simulink library "xrbsMath_r3"  (Simulink 5.0)
undefined symbols (not defined in the file or in its folder): num_width
libraries: xbsIndex_r3 x775, xrbsMath_r3 x16
(part 5 of 8)

== system xrbsMath_r3/CORDIC LOG/CORDIC Fine Angle PE/CORDIC PE4 ==
  note: X = x + y if y < 0, otherwise
      |    = x - y
      | Y = y + x if y < 0, otherwise
      |    = y - x
      | Z = z - atanh(1/2^i) if y < 0, otherwise
      |    = z + atanh(1/2^i)
  x : Inport
  y : Inport  Port=2
  z : Inport  Port=3
  AddSub : xbsIndex_r3/AddSub  mode=Addition or Subtraction  precision=User Defined  arith_type="Signed  (2's comp)"  n_bits=pe_nbits  bin_pt=pe_binpt  quantization=Truncate  overflow=Wrap  latency=pipeline  explicit_period=off  period=1  en=off  dbl_ovrd=off  use_core=on  pipeline=off  use_rpm=off  gen_core=on
      settings: xl_area=[7 14 0 14 0 0 0]
  AddSub1 : xbsIndex_r3/AddSub  mode=Addition or Subtraction  precision=User Defined  arith_type="Signed  (2's comp)"  n_bits=pe_nbits  bin_pt=pe_binpt  quantization=Truncate  overflow=Wrap  latency=pipeline  explicit_period=off  period=1  en=off  dbl_ovrd=off  use_core=on  pipeline=off  use_rpm=off  gen_core=on
      settings: xl_area=[7 14 0 14 0 0 0]
  AddSub2 : xbsIndex_r3/AddSub  mode=Addition or Subtraction  precision=User Defined  arith_type="Signed  (2's comp)"  n_bits=pe_nbits  bin_pt=pe_binpt  quantization=Truncate  overflow=Wrap  latency=pipeline  explicit_period=off  period=1  en=off  dbl_ovrd=off  use_core=on  pipeline=off  use_rpm=off  gen_core=on
      settings: xl_area=[0, 0, 0, 0, 0, 0, 0]
  Constant : xbsIndex_r3/Constant  const=atanh(1/2^ii)  arith_type="Signed  (2's comp)"  n_bits=pe_nbits  bin_pt=pe_binpt  explicit_period=off  period=1  dbl_ovrd=off
  Inverter : xbsIndex_r3/Inverter  latency=0  explicit_period=off  period=1  en=off  dbl_ovrd=off
      settings: xl_area=[1 0 0 1 0 0 0]
  Shift : xbsIndex_r3/Shift  shift_dir=Right  shift_bits=ii  precision=User Defined  arith_type="Signed  (2's comp)"  n_bits=pe_nbits  bin_pt=pe_binpt  quantization=Truncate  overflow=Wrap  latency=0  explicit_period=off  period=1  en=off  dbl_ovrd=off
      settings: xl_area=[0 0 0 0 0 0 0]
  Shift1 : xbsIndex_r3/Shift  shift_dir=Right  shift_bits=ii  precision=User Defined  arith_type="Signed  (2's comp)"  n_bits=pe_nbits  bin_pt=pe_binpt  quantization=Truncate  overflow=Wrap  latency=0  explicit_period=off  period=1  en=off  dbl_ovrd=off
      settings: xl_area=[0 0 0 0 0 0 0]
  Slice : xbsIndex_r3/Slice  mode=Upper Bit Location + Width  nbits=1  bit1=0  base1=MSB of Input  bit0=0  base0=LSB of Input  boolean_output=on  explicit_period=off  period=1  dbl_ovrd=off
  X : Outport
  Y : Outport  Port=2
  Z : Outport  Port=3
  wires:
  Constant/1 -> AddSub2/2
  AddSub2/1 -> Z/1
  z/1 -> AddSub2/1
  Slice/1 -> AddSub2/3, Inverter/1
  Shift1/1 -> AddSub/2
  Shift/1 -> AddSub1/2
  AddSub1/1 -> Y/1
  AddSub/1 -> X/1
  y/1 -> Slice/1, Shift1/1, AddSub1/1
  x/1 -> Shift/1, AddSub/1
  Inverter/1 -> AddSub/3, AddSub1/3

== system xrbsMath_r3/CORDIC LOG/CORDIC Fine Angle PE/CORDIC PE5 ==
  note: X = x + y if y < 0, otherwise
      |    = x - y
      | Y = y + x if y < 0, otherwise
      |    = y - x
      | Z = z - atanh(1/2^i) if y < 0, otherwise
      |    = z + atanh(1/2^i)
  x : Inport
  y : Inport  Port=2
  z : Inport  Port=3
  AddSub : xbsIndex_r3/AddSub  mode=Addition or Subtraction  precision=User Defined  arith_type="Signed  (2's comp)"  n_bits=pe_nbits  bin_pt=pe_binpt  quantization=Truncate  overflow=Wrap  latency=pipeline  explicit_period=off  period=1  en=off  dbl_ovrd=off  use_core=on  pipeline=off  use_rpm=off  gen_core=on
      settings: xl_area=[7 14 0 14 0 0 0]
  AddSub1 : xbsIndex_r3/AddSub  mode=Addition or Subtraction  precision=User Defined  arith_type="Signed  (2's comp)"  n_bits=pe_nbits  bin_pt=pe_binpt  quantization=Truncate  overflow=Wrap  latency=pipeline  explicit_period=off  period=1  en=off  dbl_ovrd=off  use_core=on  pipeline=off  use_rpm=off  gen_core=on
      settings: xl_area=[7 14 0 14 0 0 0]
  AddSub2 : xbsIndex_r3/AddSub  mode=Addition or Subtraction  precision=User Defined  arith_type="Signed  (2's comp)"  n_bits=pe_nbits  bin_pt=pe_binpt  quantization=Truncate  overflow=Wrap  latency=pipeline  explicit_period=off  period=1  en=off  dbl_ovrd=off  use_core=on  pipeline=off  use_rpm=off  gen_core=on
      settings: xl_area=[0, 0, 0, 0, 0, 0, 0]
  Constant : xbsIndex_r3/Constant  const=atanh(1/2^ii)  arith_type="Signed  (2's comp)"  n_bits=pe_nbits  bin_pt=pe_binpt  explicit_period=off  period=1  dbl_ovrd=off
  Inverter : xbsIndex_r3/Inverter  latency=0  explicit_period=off  period=1  en=off  dbl_ovrd=off
      settings: xl_area=[1 0 0 1 0 0 0]
  Shift : xbsIndex_r3/Shift  shift_dir=Right  shift_bits=ii  precision=User Defined  arith_type="Signed  (2's comp)"  n_bits=pe_nbits  bin_pt=pe_binpt  quantization=Truncate  overflow=Wrap  latency=0  explicit_period=off  period=1  en=off  dbl_ovrd=off
      settings: xl_area=[0 0 0 0 0 0 0]
  Shift1 : xbsIndex_r3/Shift  shift_dir=Right  shift_bits=ii  precision=User Defined  arith_type="Signed  (2's comp)"  n_bits=pe_nbits  bin_pt=pe_binpt  quantization=Truncate  overflow=Wrap  latency=0  explicit_period=off  period=1  en=off  dbl_ovrd=off
      settings: xl_area=[0 0 0 0 0 0 0]
  Slice : xbsIndex_r3/Slice  mode=Upper Bit Location + Width  nbits=1  bit1=0  base1=MSB of Input  bit0=0  base0=LSB of Input  boolean_output=on  explicit_period=off  period=1  dbl_ovrd=off
  X : Outport
  Y : Outport  Port=2
  Z : Outport  Port=3
  wires:
  Constant/1 -> AddSub2/2
  AddSub2/1 -> Z/1
  z/1 -> AddSub2/1
  Slice/1 -> AddSub2/3, Inverter/1
  Shift1/1 -> AddSub/2
  Shift/1 -> AddSub1/2
  AddSub1/1 -> Y/1
  AddSub/1 -> X/1
  y/1 -> Slice/1, Shift1/1, AddSub1/1
  x/1 -> Shift/1, AddSub/1
  Inverter/1 -> AddSub/3, AddSub1/3

== system xrbsMath_r3/CORDIC LOG/CORDIC Fine Angle PE/CORDIC PE6 ==
  note: X = x + y if y < 0, otherwise
      |    = x - y
      | Y = y + x if y < 0, otherwise
      |    = y - x
      | Z = z - atanh(1/2^i) if y < 0, otherwise
      |    = z + atanh(1/2^i)
  x : Inport
  y : Inport  Port=2
  z : Inport  Port=3
  AddSub : xbsIndex_r3/AddSub  mode=Addition or Subtraction  precision=User Defined  arith_type="Signed  (2's comp)"  n_bits=pe_nbits  bin_pt=pe_binpt  quantization=Truncate  overflow=Wrap  latency=pipeline  explicit_period=off  period=1  en=off  dbl_ovrd=off  use_core=on  pipeline=off  use_rpm=off  gen_core=on
      settings: xl_area=[7 14 0 14 0 0 0]
  AddSub1 : xbsIndex_r3/AddSub  mode=Addition or Subtraction  precision=User Defined  arith_type="Signed  (2's comp)"  n_bits=pe_nbits  bin_pt=pe_binpt  quantization=Truncate  overflow=Wrap  latency=pipeline  explicit_period=off  period=1  en=off  dbl_ovrd=off  use_core=on  pipeline=off  use_rpm=off  gen_core=on
      settings: xl_area=[7 14 0 14 0 0 0]
  AddSub2 : xbsIndex_r3/AddSub  mode=Addition or Subtraction  precision=User Defined  arith_type="Signed  (2's comp)"  n_bits=pe_nbits  bin_pt=pe_binpt  quantization=Truncate  overflow=Wrap  latency=pipeline  explicit_period=off  period=1  en=off  dbl_ovrd=off  use_core=on  pipeline=off  use_rpm=off  gen_core=on
      settings: xl_area=[0, 0, 0, 0, 0, 0, 0]
  Constant : xbsIndex_r3/Constant  const=atanh(1/2^ii)  arith_type="Signed  (2's comp)"  n_bits=pe_nbits  bin_pt=pe_binpt  explicit_period=off  period=1  dbl_ovrd=off
  Inverter : xbsIndex_r3/Inverter  latency=0  explicit_period=off  period=1  en=off  dbl_ovrd=off
      settings: xl_area=[1 0 0 1 0 0 0]
  Shift : xbsIndex_r3/Shift  shift_dir=Right  shift_bits=ii  precision=User Defined  arith_type="Signed  (2's comp)"  n_bits=pe_nbits  bin_pt=pe_binpt  quantization=Truncate  overflow=Wrap  latency=0  explicit_period=off  period=1  en=off  dbl_ovrd=off
      settings: xl_area=[0 0 0 0 0 0 0]
  Shift1 : xbsIndex_r3/Shift  shift_dir=Right  shift_bits=ii  precision=User Defined  arith_type="Signed  (2's comp)"  n_bits=pe_nbits  bin_pt=pe_binpt  quantization=Truncate  overflow=Wrap  latency=0  explicit_period=off  period=1  en=off  dbl_ovrd=off
      settings: xl_area=[0 0 0 0 0 0 0]
  Slice : xbsIndex_r3/Slice  mode=Upper Bit Location + Width  nbits=1  bit1=0  base1=MSB of Input  bit0=0  base0=LSB of Input  boolean_output=on  explicit_period=off  period=1  dbl_ovrd=off
  X : Outport
  Y : Outport  Port=2
  Z : Outport  Port=3
  wires:
  Constant/1 -> AddSub2/2
  AddSub2/1 -> Z/1
  z/1 -> AddSub2/1
  Slice/1 -> AddSub2/3, Inverter/1
  Shift1/1 -> AddSub/2
  Shift/1 -> AddSub1/2
  AddSub1/1 -> Y/1
  AddSub/1 -> X/1
  y/1 -> Slice/1, Shift1/1, AddSub1/1
  x/1 -> Shift/1, AddSub/1
  Inverter/1 -> AddSub/3, AddSub1/3

== system xrbsMath_r3/CORDIC LOG/CORDIC Fine Angle PE/CORDIC PE7 ==
  note: X = x + y if y < 0, otherwise
      |    = x - y
      | Y = y + x if y < 0, otherwise
      |    = y - x
      | Z = z - atanh(1/2^i) if y < 0, otherwise
      |    = z + atanh(1/2^i)
  x : Inport
  y : Inport  Port=2
  z : Inport  Port=3
  AddSub : xbsIndex_r3/AddSub  mode=Addition or Subtraction  precision=User Defined  arith_type="Signed  (2's comp)"  n_bits=pe_nbits  bin_pt=pe_binpt  quantization=Truncate  overflow=Wrap  latency=pipeline  explicit_period=off  period=1  en=off  dbl_ovrd=off  use_core=on  pipeline=off  use_rpm=off  gen_core=on
      settings: xl_area=[7 14 0 14 0 0 0]
  AddSub1 : xbsIndex_r3/AddSub  mode=Addition or Subtraction  precision=User Defined  arith_type="Signed  (2's comp)"  n_bits=pe_nbits  bin_pt=pe_binpt  quantization=Truncate  overflow=Wrap  latency=pipeline  explicit_period=off  period=1  en=off  dbl_ovrd=off  use_core=on  pipeline=off  use_rpm=off  gen_core=on
      settings: xl_area=[7 14 0 14 0 0 0]
  AddSub2 : xbsIndex_r3/AddSub  mode=Addition or Subtraction  precision=User Defined  arith_type="Signed  (2's comp)"  n_bits=pe_nbits  bin_pt=pe_binpt  quantization=Truncate  overflow=Wrap  latency=pipeline  explicit_period=off  period=1  en=off  dbl_ovrd=off  use_core=on  pipeline=off  use_rpm=off  gen_core=on
      settings: xl_area=[0, 0, 0, 0, 0, 0, 0]
  Constant : xbsIndex_r3/Constant  const=atanh(1/2^ii)  arith_type="Signed  (2's comp)"  n_bits=pe_nbits  bin_pt=pe_binpt  explicit_period=off  period=1  dbl_ovrd=off
  Inverter : xbsIndex_r3/Inverter  latency=0  explicit_period=off  period=1  en=off  dbl_ovrd=off
      settings: xl_area=[1 0 0 1 0 0 0]
  Shift : xbsIndex_r3/Shift  shift_dir=Right  shift_bits=ii  precision=User Defined  arith_type="Signed  (2's comp)"  n_bits=pe_nbits  bin_pt=pe_binpt  quantization=Truncate  overflow=Wrap  latency=0  explicit_period=off  period=1  en=off  dbl_ovrd=off
      settings: xl_area=[0 0 0 0 0 0 0]
  Shift1 : xbsIndex_r3/Shift  shift_dir=Right  shift_bits=ii  precision=User Defined  arith_type="Signed  (2's comp)"  n_bits=pe_nbits  bin_pt=pe_binpt  quantization=Truncate  overflow=Wrap  latency=0  explicit_period=off  period=1  en=off  dbl_ovrd=off
      settings: xl_area=[0 0 0 0 0 0 0]
  Slice : xbsIndex_r3/Slice  mode=Upper Bit Location + Width  nbits=1  bit1=0  base1=MSB of Input  bit0=0  base0=LSB of Input  boolean_output=on  explicit_period=off  period=1  dbl_ovrd=off
  X : Outport
  Y : Outport  Port=2
  Z : Outport  Port=3
  wires:
  Constant/1 -> AddSub2/2
  AddSub2/1 -> Z/1
  z/1 -> AddSub2/1
  Slice/1 -> AddSub2/3, Inverter/1
  Shift1/1 -> AddSub/2
  Shift/1 -> AddSub1/2
  AddSub1/1 -> Y/1
  AddSub/1 -> X/1
  y/1 -> Slice/1, Shift1/1, AddSub1/1
  x/1 -> Shift/1, AddSub/1
  Inverter/1 -> AddSub/3, AddSub1/3

== system xrbsMath_r3/CORDIC LOG/CORDIC Fine Angle PE/CORDIC PE8 ==
  note: X = x + y if y < 0, otherwise
      |    = x - y
      | Y = y + x if y < 0, otherwise
      |    = y - x
      | Z = z - atanh(1/2^i) if y < 0, otherwise
      |    = z + atanh(1/2^i)
  x : Inport
  y : Inport  Port=2
  z : Inport  Port=3
  AddSub : xbsIndex_r3/AddSub  mode=Addition or Subtraction  precision=User Defined  arith_type="Signed  (2's comp)"  n_bits=pe_nbits  bin_pt=pe_binpt  quantization=Truncate  overflow=Wrap  latency=pipeline  explicit_period=off  period=1  en=off  dbl_ovrd=off  use_core=on  pipeline=off  use_rpm=off  gen_core=on
      settings: xl_area=[7 14 0 14 0 0 0]
  AddSub1 : xbsIndex_r3/AddSub  mode=Addition or Subtraction  precision=User Defined  arith_type="Signed  (2's comp)"  n_bits=pe_nbits  bin_pt=pe_binpt  quantization=Truncate  overflow=Wrap  latency=pipeline  explicit_period=off  period=1  en=off  dbl_ovrd=off  use_core=on  pipeline=off  use_rpm=off  gen_core=on
      settings: xl_area=[7 14 0 14 0 0 0]
  AddSub2 : xbsIndex_r3/AddSub  mode=Addition or Subtraction  precision=User Defined  arith_type="Signed  (2's comp)"  n_bits=pe_nbits  bin_pt=pe_binpt  quantization=Truncate  overflow=Wrap  latency=pipeline  explicit_period=off  period=1  en=off  dbl_ovrd=off  use_core=on  pipeline=off  use_rpm=off  gen_core=on
      settings: xl_area=[0, 0, 0, 0, 0, 0, 0]
  Constant : xbsIndex_r3/Constant  const=atanh(1/2^ii)  arith_type="Signed  (2's comp)"  n_bits=pe_nbits  bin_pt=pe_binpt  explicit_period=off  period=1  dbl_ovrd=off
  Inverter : xbsIndex_r3/Inverter  latency=0  explicit_period=off  period=1  en=off  dbl_ovrd=off
      settings: xl_area=[1 0 0 1 0 0 0]
  Shift : xbsIndex_r3/Shift  shift_dir=Right  shift_bits=ii  precision=User Defined  arith_type="Signed  (2's comp)"  n_bits=pe_nbits  bin_pt=pe_binpt  quantization=Truncate  overflow=Wrap  latency=0  explicit_period=off  period=1  en=off  dbl_ovrd=off
      settings: xl_area=[0 0 0 0 0 0 0]
  Shift1 : xbsIndex_r3/Shift  shift_dir=Right  shift_bits=ii  precision=User Defined  arith_type="Signed  (2's comp)"  n_bits=pe_nbits  bin_pt=pe_binpt  quantization=Truncate  overflow=Wrap  latency=0  explicit_period=off  period=1  en=off  dbl_ovrd=off
      settings: xl_area=[0 0 0 0 0 0 0]
  Slice : xbsIndex_r3/Slice  mode=Upper Bit Location + Width  nbits=1  bit1=0  base1=MSB of Input  bit0=0  base0=LSB of Input  boolean_output=on  explicit_period=off  period=1  dbl_ovrd=off
  X : Outport
  Y : Outport  Port=2
  Z : Outport  Port=3
  wires:
  Constant/1 -> AddSub2/2
  AddSub2/1 -> Z/1
  z/1 -> AddSub2/1
  Slice/1 -> AddSub2/3, Inverter/1
  Shift1/1 -> AddSub/2
  Shift/1 -> AddSub1/2
  AddSub1/1 -> Y/1
  AddSub/1 -> X/1
  y/1 -> Slice/1, Shift1/1, AddSub1/1
  x/1 -> Shift/1, AddSub/1
  Inverter/1 -> AddSub/3, AddSub1/3

== system xrbsMath_r3/CORDIC LOG/Quadrant Map/Co-ordinate Correction ==
  x : Inport
  Constant3 : xbsIndex_r3/Constant  const=0  arith_type=Unsigned  n_bits=1  bin_pt=0  explicit_period=off  period=1  dbl_ovrd=off
  Delay4 : xbsIndex_r3/Delay  latency=1  reg_retiming=off  explicit_period=off  period=1  en=off  accept_only_valid=off  init_zero=on  dbl_ovrd=off
      settings: xl_area=[6 12 0 0 0 0 0]
  Mux : xbsIndex_r3/Mux  inputs=2  precision=User Defined  arith_type="Signed  (2's comp)"  n_bits=pe_nbits  bin_pt=pe_binpt  quantization=Truncate  overflow=Wrap  latency=1  mux_type=off  explicit_period=off  period=1  en=off  dbl_ovrd=off  use_rpm=off  gen_core=on
      settings: xl_area=[6 12 0 12 0 0 0]
  Negate1 : xbsIndex_r3/Negate  precision=User Defined  arith_type="Signed  (2's comp)"  n_bits=pe_nbits  bin_pt=pe_binpt  quantization=Truncate  overflow=Wrap  latency=0  explicit_period=off  period=1  en=off  dbl_ovrd=off  use_core=on  use_rpm=off  gen_core=on
      settings: xl_area=[6 0 0 12 0 0 0]
  Reinterpret : xbsIndex_r3/Reinterpret  force_arith_type=off  arith_type="Signed  (2's comp)"  force_bin_pt=on  bin_pt=pe_nbits-1  force_valid=on
  Relational : xbsIndex_r3/Relational  mode=a=b  latency=1  explicit_period=off  period=1  en=off  dbl_ovrd=off
      settings: xl_area=[3 0 0 6 0 0 0]
  sgn(x) : xbsIndex_r3/Slice  mode=Upper Bit Location + Width  nbits=1  bit1=0  base1=MSB of Input  bit0=0  base0=LSB of Input  boolean_output=off  explicit_period=off  period=1  dbl_ovrd=off
  X : Outport
  sign_x : Outport  Port=2
  zero_detect : Outport  Port=3
  wires:
  Relational/1 -> zero_detect/1
  x/1 -> Delay4/1
  Constant3/1 -> Relational/2
  Reinterpret/1 -> X/1
  Mux/1 -> Reinterpret/1
  Negate1/1 -> Mux/3
  sgn(x)/1 -> sign_x/1, Mux/1
  Delay4/1 -> Relational/1, sgn(x)/1, Negate1/1, Mux/2

== system xrbsMath_r3/CORDIC LOG/Quadrant Map/Normalize X ==
  note: Normalizing X : The absolute value of X is shifted left till we have a 1
      | on the most significant bit and the number of shifts are recorded.
  abs : Inport
  cin : Inport  Port=2
  msb : Inport  Port=3
  Shift1 : Subsystem  mask(Normalize Shift Stage){num_bits=num_bits, bin_point=bin_point}
      mask prompts: num_bits "Number of Bits"; bin_point "Binary Point Position"
      mask init:
      | [bg,fg] = xlcmap('XBlock',0);
      | iPos = get_param(gcb,'Position');
      | iWidth=iPos(3)-iPos(1); iHeight=iPos(4)-iPos(2);
      | iCx=iWidth/2;
      | iCy=iHeight/2;
      | [logoX, logoY] = xlogo(iPos);
      mask Display:
      | patch([0 iWidth iWidth 0],[0 0 iHeight iHeight] , bg);
      | patch(logoX,logoY , fg);
      | port_label('input',1,'din');
      | port_label('input',2,'cin');
      | port_label('input',3,'msb');
      | port_label('output',1,'dout');
      | port_label('output',2,'sum');
      | port_label('output',3,'latch');
      | plot([0 0 iWidth iWidth 0], [0 iHeight iHeight 0 0]);
  Shift{2..7} (6 alike) : xrbsMath_r3/CORDIC LOG/Quadrant Map/Normalize X/Shift1  num_bits=num_bits  bin_point=bin_point
  Terminator1 : Terminator
  norm : Outport
  shift : Outport  Port=2
  wires:
  abs/1 -> Shift1/1(din)
  cin/1 -> Shift1/2(cin)
  msb/1 -> Shift1/3(msb)
  Shift1/1(dout) -> Shift2/1
  Shift1/2(sum) -> Shift2/2
  Shift1/3(latch) -> Shift2/3
  Shift2/1 -> Shift3/1
  Shift2/2 -> Shift3/2
  Shift2/3 -> Shift3/3
  Shift3/1 -> Shift4/1
  Shift3/2 -> Shift4/2
  Shift3/3 -> Shift4/3
  Shift4/1 -> Shift5/1
  Shift4/2 -> Shift5/2
  Shift4/3 -> Shift5/3
  Shift5/1 -> Shift6/1
  Shift5/2 -> Shift6/2
  Shift5/3 -> Shift6/3
  Shift6/1 -> Shift7/1
  Shift6/2 -> Shift7/2
  Shift6/3 -> Shift7/3
  Shift7/1 -> norm/1
  Shift7/2 -> shift/1
  Shift7/3 -> Terminator1/1

== system xrbsMath_r3/CORDIC LOG/Quadrant Map/Post Normalization ==
  norm_x : Inport
  shift_in : Inport  Port=2
  AddSub1 : xbsIndex_r3/AddSub  mode=Addition  precision=User Defined  arith_type="Signed  (2's comp)"  n_bits=pe_nbits+1  bin_pt=pe_nbits-1  quantization=Truncate  overflow=Wrap  latency=0  explicit_period=off  period=1  en=off  dbl_ovrd=off  use_core=on  pipeline=off  use_rpm=off  gen_core=off
      settings: xl_area=[7 0 0 14 0 0 0]
  AddSub2 : xbsIndex_r3/AddSub  mode=Subtraction  precision=User Defined  arith_type="Signed  (2's comp)"  n_bits=pe_nbits+1  bin_pt=pe_nbits-1  quantization=Truncate  overflow=Wrap  latency=0  explicit_period=off  period=1  en=off  dbl_ovrd=off  use_core=on  pipeline=off  use_rpm=off  gen_core=off
      settings: xl_area=[7 0 0 14 0 0 0]
  Constant2 : xbsIndex_r3/Constant  const=1  arith_type=Unsigned  n_bits=1  bin_pt=0  explicit_period=off  period=1  dbl_ovrd=off
  Constant4 : xbsIndex_r3/Constant  const=0  arith_type="Signed  (2's comp)"  n_bits=pe_nbits+1  bin_pt=pe_nbits-1  explicit_period=off  period=1  dbl_ovrd=off
  Slice1 : xbsIndex_r3/Slice  mode=Lower Bit Location + Width  nbits=ceil(log2(pe_nbits))  bit1=0  base1=MSB of Input  bit0=0  base0=LSB of Input  boolean_output=off  explicit_period=off  period=1  dbl_ovrd=off
  X : Outport
  Y : Outport  Port=2
  Z : Outport  Port=3
  shift_out : Outport  Port=4
  wires:
  Constant4/1 -> Z/1
  Slice1/1 -> shift_out/1
  shift_in/1 -> Slice1/1
  AddSub2/1 -> Y/1
  AddSub1/1 -> X/1
  Constant2/1 -> AddSub2/2, AddSub1/2
  norm_x/1 -> AddSub2/1, AddSub1/1

== system xrbsMath_r3/CORDIC SINCOS/CORDIC Fine Angle PE/CORDIC PE1 ==
  note: X = x + y if z < 0, otherwise
      |    = x - y
      | Y = y - x if z < 0, otherwise
      |    = y + x
      | Z = z + atan(1/2^i) if z < 0, otherwise
      |    = z - atan(1/2^i)
  x : Inport
  y : Inport  Port=2
  z : Inport  Port=3
  AddSub : xbsIndex_r3/AddSub  mode=Addition or Subtraction  precision=User Defined  arith_type="Signed  (2's comp)"  n_bits=pe_nbits  bin_pt=pe_binpt  quantization=Truncate  overflow=Wrap  latency=pipeline  explicit_period=off  period=1  en=off  dbl_ovrd=off  use_core=on  pipeline=off  use_rpm=off  gen_core=on
      settings: xl_area=[8 16 0 16 0 0 0]
  AddSub1 : xbsIndex_r3/AddSub  mode=Addition or Subtraction  precision=User Defined  arith_type="Signed  (2's comp)"  n_bits=pe_nbits  bin_pt=pe_binpt  quantization=Truncate  overflow=Wrap  latency=pipeline  explicit_period=off  period=1  en=off  dbl_ovrd=off  use_core=on  pipeline=off  use_rpm=off  gen_core=on
      settings: xl_area=[8 16 0 16 0 0 0]
  AddSub2 : xbsIndex_r3/AddSub  mode=Addition or Subtraction  precision=User Defined  arith_type="Signed  (2's comp)"  n_bits=pe_nbits  bin_pt=pe_binpt  quantization=Truncate  overflow=Wrap  latency=pipeline  explicit_period=off  period=1  en=off  dbl_ovrd=off  use_core=on  pipeline=off  use_rpm=off  gen_core=on
      settings: xl_area=[8 16 0 16 0 0 0]
  Constant : xbsIndex_r3/Constant  const=epsilon_k  arith_type="Signed  (2's comp)"  n_bits=pe_nbits  bin_pt=pe_binpt  explicit_period=off  period=1  dbl_ovrd=off
  Inverter : xbsIndex_r3/Inverter  latency=0  explicit_period=off  period=1  en=off  dbl_ovrd=off
      settings: xl_area=[1 0 0 1 0 0 0]
  Shift : xbsIndex_r3/Shift  shift_dir=Right  shift_bits=ii  precision=User Defined  arith_type="Signed  (2's comp)"  n_bits=pe_nbits  bin_pt=pe_binpt  quantization=Truncate  overflow=Wrap  latency=0  explicit_period=off  period=1  en=off  dbl_ovrd=off
      settings: xl_area=[0 0 0 0 0 0 0]
  Shift1 : xbsIndex_r3/Shift  shift_dir=Right  shift_bits=ii  precision=User Defined  arith_type="Signed  (2's comp)"  n_bits=pe_nbits  bin_pt=pe_binpt  quantization=Truncate  overflow=Wrap  latency=0  explicit_period=off  period=1  en=off  dbl_ovrd=off
      settings: xl_area=[0 0 0 0 0 0 0]
  Slice : xbsIndex_r3/Slice  mode=Upper Bit Location + Width  nbits=1  bit1=0  base1=MSB of Input  bit0=0  base0=LSB of Input  boolean_output=on  explicit_period=off  period=1  dbl_ovrd=off
  X : Outport
  Y : Outport  Port=2
  Z : Outport  Port=3
  wires:
  Inverter/1 -> AddSub/3, AddSub2/3
  Slice/1 -> AddSub1/3, Inverter/1
  Shift1/1 -> AddSub/2
  Shift/1 -> AddSub1/2
  Constant/1 -> AddSub2/2
  AddSub2/1 -> Z/1
  AddSub1/1 -> Y/1
  z/1 -> Slice/1, AddSub2/1
  AddSub/1 -> X/1
  y/1 -> Shift1/1, AddSub1/1
  x/1 -> Shift/1, AddSub/1

== system xrbsMath_r3/CORDIC SINCOS/CORDIC Fine Angle PE/CORDIC PE2 ==
  note: X = x + y if z < 0, otherwise
      |    = x - y
      | Y = y - x if z < 0, otherwise
      |    = y + x
      | Z = z + atan(1/2^i) if z < 0, otherwise
      |    = z - atan(1/2^i)
  x : Inport
  y : Inport  Port=2
  z : Inport  Port=3
  AddSub : xbsIndex_r3/AddSub  mode=Addition or Subtraction  precision=User Defined  arith_type="Signed  (2's comp)"  n_bits=pe_nbits  bin_pt=pe_binpt  quantization=Truncate  overflow=Wrap  latency=pipeline  explicit_period=off  period=1  use_carryin=off  use_carryout=off  en=off  dbl_ovrd=off  show_param=off  use_core=on  pipeline=off  use_rpm=off  gen_core=on
      settings: xl_area=[8 16 0 16 0 0 0]
  AddSub1 : xbsIndex_r3/AddSub  mode=Addition or Subtraction  precision=User Defined  arith_type="Signed  (2's comp)"  n_bits=pe_nbits  bin_pt=pe_binpt  quantization=Truncate  overflow=Wrap  latency=pipeline  explicit_period=off  period=1  use_carryin=off  use_carryout=off  en=off  dbl_ovrd=off  show_param=off  use_core=on  pipeline=off  use_rpm=off  gen_core=on
      settings: xl_area=[8 16 0 16 0 0 0]
  AddSub2 : xbsIndex_r3/AddSub  mode=Addition or Subtraction  precision=User Defined  arith_type="Signed  (2's comp)"  n_bits=pe_nbits  bin_pt=pe_binpt  quantization=Truncate  overflow=Wrap  latency=pipeline  explicit_period=off  period=1  use_carryin=off  use_carryout=off  en=off  dbl_ovrd=off  show_param=off  use_core=on  pipeline=off  use_rpm=off  gen_core=on
      settings: xl_area=[8 16 0 16 0 0 0]
  Constant : xbsIndex_r3/Constant  const=epsilon_k  arith_type="Signed  (2's comp)"  n_bits=pe_nbits  bin_pt=pe_binpt  explicit_period=off  period=1  dbl_ovrd=off
  Inverter : xbsIndex_r3/Inverter  latency=0  explicit_period=off  period=1  en=off  dbl_ovrd=off  show_param=off
      settings: xl_area=[1 0 0 1 0 0 0]
  Shift : xbsIndex_r3/Shift  shift_dir=Right  shift_bits=ii  precision=User Defined  arith_type="Signed  (2's comp)"  n_bits=pe_nbits  bin_pt=pe_binpt  quantization=Truncate  overflow=Wrap  latency=0  explicit_period=off  period=1  en=off  dbl_ovrd=off  show_param=off
      settings: xl_area=[0 0 0 0 0 0 0]
  Shift1 : xbsIndex_r3/Shift  shift_dir=Right  shift_bits=ii  precision=User Defined  arith_type="Signed  (2's comp)"  n_bits=pe_nbits  bin_pt=pe_binpt  quantization=Truncate  overflow=Wrap  latency=0  explicit_period=off  period=1  en=off  dbl_ovrd=off  show_param=off
      settings: xl_area=[0 0 0 0 0 0 0]
  Slice : xbsIndex_r3/Slice  mode=Upper Bit Location + Width  nbits=1  bit1=0  base1=MSB of Input  bit0=0  base0=LSB of Input  boolean_output=on  explicit_period=off  period=1  dbl_ovrd=off
  X : Outport
  Y : Outport  Port=2
  Z : Outport  Port=3
  wires:
  x/1 -> AddSub/1, Shift/1
  y/1 -> AddSub1/1, Shift1/1
  AddSub/1 -> X/1
  z/1 -> AddSub2/1, Slice/1
  AddSub1/1 -> Y/1
  AddSub2/1 -> Z/1
  Constant/1 -> AddSub2/2
  Shift/1 -> AddSub1/2
  Shift1/1 -> AddSub/2
  Slice/1 -> Inverter/1, AddSub1/3
  Inverter/1 -> AddSub2/3, AddSub/3

== system xrbsMath_r3/CORDIC SINCOS/CORDIC Fine Angle PE/CORDIC PE3 ==
  note: X = x + y if z < 0, otherwise
      |    = x - y
      | Y = y - x if z < 0, otherwise
      |    = y + x
      | Z = z + atan(1/2^i) if z < 0, otherwise
      |    = z - atan(1/2^i)
  x : Inport
  y : Inport  Port=2
  z : Inport  Port=3
  AddSub : xbsIndex_r3/AddSub  mode=Addition or Subtraction  precision=User Defined  arith_type="Signed  (2's comp)"  n_bits=pe_nbits  bin_pt=pe_binpt  quantization=Truncate  overflow=Wrap  latency=pipeline  explicit_period=off  period=1  en=off  dbl_ovrd=off  use_core=on  pipeline=off  use_rpm=off  gen_core=on
      settings: xl_area=[8 16 0 16 0 0 0]
  AddSub1 : xbsIndex_r3/AddSub  mode=Addition or Subtraction  precision=User Defined  arith_type="Signed  (2's comp)"  n_bits=pe_nbits  bin_pt=pe_binpt  quantization=Truncate  overflow=Wrap  latency=pipeline  explicit_period=off  period=1  en=off  dbl_ovrd=off  use_core=on  pipeline=off  use_rpm=off  gen_core=on
      settings: xl_area=[8 16 0 16 0 0 0]
  AddSub2 : xbsIndex_r3/AddSub  mode=Addition or Subtraction  precision=User Defined  arith_type="Signed  (2's comp)"  n_bits=pe_nbits  bin_pt=pe_binpt  quantization=Truncate  overflow=Wrap  latency=pipeline  explicit_period=off  period=1  en=off  dbl_ovrd=off  use_core=on  pipeline=off  use_rpm=off  gen_core=on
      settings: xl_area=[8 16 0 16 0 0 0]
  Constant : xbsIndex_r3/Constant  const=epsilon_k  arith_type="Signed  (2's comp)"  n_bits=pe_nbits  bin_pt=pe_binpt  explicit_period=off  period=1  dbl_ovrd=off
  Inverter : xbsIndex_r3/Inverter  latency=0  explicit_period=off  period=1  en=off  dbl_ovrd=off
      settings: xl_area=[1 0 0 1 0 0 0]
  Shift : xbsIndex_r3/Shift  shift_dir=Right  shift_bits=ii  precision=User Defined  arith_type="Signed  (2's comp)"  n_bits=pe_nbits  bin_pt=pe_binpt  quantization=Truncate  overflow=Wrap  latency=0  explicit_period=off  period=1  en=off  dbl_ovrd=off
      settings: xl_area=[0 0 0 0 0 0 0]
  Shift1 : xbsIndex_r3/Shift  shift_dir=Right  shift_bits=ii  precision=User Defined  arith_type="Signed  (2's comp)"  n_bits=pe_nbits  bin_pt=pe_binpt  quantization=Truncate  overflow=Wrap  latency=0  explicit_period=off  period=1  en=off  dbl_ovrd=off
      settings: xl_area=[0 0 0 0 0 0 0]
  Slice : xbsIndex_r3/Slice  mode=Upper Bit Location + Width  nbits=1  bit1=0  base1=MSB of Input  bit0=0  base0=LSB of Input  boolean_output=on  explicit_period=off  period=1  dbl_ovrd=off
  X : Outport
  Y : Outport  Port=2
  Z : Outport  Port=3
  wires:
  x/1 -> AddSub/1, Shift/1
  y/1 -> AddSub1/1, Shift1/1
  AddSub/1 -> X/1
  z/1 -> AddSub2/1, Slice/1
  AddSub1/1 -> Y/1
  AddSub2/1 -> Z/1
  Constant/1 -> AddSub2/2
  Shift/1 -> AddSub1/2
  Shift1/1 -> AddSub/2
  Slice/1 -> Inverter/1, AddSub1/3
  Inverter/1 -> AddSub2/3, AddSub/3

== system xrbsMath_r3/CORDIC SINCOS/CORDIC Fine Angle PE/CORDIC PE4 ==
  note: X = x + y if z < 0, otherwise
      |    = x - y
      | Y = y - x if z < 0, otherwise
      |    = y + x
      | Z = z + atan(1/2^i) if z < 0, otherwise
      |    = z - atan(1/2^i)
  x : Inport
  y : Inport  Port=2
  z : Inport  Port=3
  AddSub : xbsIndex_r3/AddSub  mode=Addition or Subtraction  precision=User Defined  arith_type="Signed  (2's comp)"  n_bits=pe_nbits  bin_pt=pe_binpt  quantization=Truncate  overflow=Wrap  latency=pipeline  explicit_period=off  period=1  en=off  dbl_ovrd=off  use_core=on  pipeline=off  use_rpm=off  gen_core=on
      settings: xl_area=[8 16 0 16 0 0 0]
  AddSub1 : xbsIndex_r3/AddSub  mode=Addition or Subtraction  precision=User Defined  arith_type="Signed  (2's comp)"  n_bits=pe_nbits  bin_pt=pe_binpt  quantization=Truncate  overflow=Wrap  latency=pipeline  explicit_period=off  period=1  en=off  dbl_ovrd=off  use_core=on  pipeline=off  use_rpm=off  gen_core=on
      settings: xl_area=[8 16 0 16 0 0 0]
  AddSub2 : xbsIndex_r3/AddSub  mode=Addition or Subtraction  precision=User Defined  arith_type="Signed  (2's comp)"  n_bits=pe_nbits  bin_pt=pe_binpt  quantization=Truncate  overflow=Wrap  latency=pipeline  explicit_period=off  period=1  en=off  dbl_ovrd=off  use_core=on  pipeline=off  use_rpm=off  gen_core=on
      settings: xl_area=[8 16 0 16 0 0 0]
  Constant : xbsIndex_r3/Constant  const=epsilon_k  arith_type="Signed  (2's comp)"  n_bits=pe_nbits  bin_pt=pe_binpt  explicit_period=off  period=1  dbl_ovrd=off
  Inverter : xbsIndex_r3/Inverter  latency=0  explicit_period=off  period=1  en=off  dbl_ovrd=off
      settings: xl_area=[1 0 0 1 0 0 0]
  Shift : xbsIndex_r3/Shift  shift_dir=Right  shift_bits=ii  precision=User Defined  arith_type="Signed  (2's comp)"  n_bits=pe_nbits  bin_pt=pe_binpt  quantization=Truncate  overflow=Wrap  latency=0  explicit_period=off  period=1  en=off  dbl_ovrd=off
      settings: xl_area=[0 0 0 0 0 0 0]
  Shift1 : xbsIndex_r3/Shift  shift_dir=Right  shift_bits=ii  precision=User Defined  arith_type="Signed  (2's comp)"  n_bits=pe_nbits  bin_pt=pe_binpt  quantization=Truncate  overflow=Wrap  latency=0  explicit_period=off  period=1  en=off  dbl_ovrd=off
      settings: xl_area=[0 0 0 0 0 0 0]
  Slice : xbsIndex_r3/Slice  mode=Upper Bit Location + Width  nbits=1  bit1=0  base1=MSB of Input  bit0=0  base0=LSB of Input  boolean_output=on  explicit_period=off  period=1  dbl_ovrd=off
  X : Outport
  Y : Outport  Port=2
  Z : Outport  Port=3
  wires:
  x/1 -> AddSub/1, Shift/1
  y/1 -> AddSub1/1, Shift1/1
  AddSub/1 -> X/1
  z/1 -> AddSub2/1, Slice/1
  AddSub1/1 -> Y/1
  AddSub2/1 -> Z/1
  Constant/1 -> AddSub2/2
  Shift/1 -> AddSub1/2
  Shift1/1 -> AddSub/2
  Slice/1 -> Inverter/1, AddSub1/3
  Inverter/1 -> AddSub2/3, AddSub/3

== system xrbsMath_r3/CORDIC SINCOS/CORDIC Fine Angle PE/CORDIC PE5 ==
  note: X = x + y if z < 0, otherwise
      |    = x - y
      | Y = y - x if z < 0, otherwise
      |    = y + x
      | Z = z + atan(1/2^i) if z < 0, otherwise
      |    = z - atan(1/2^i)
  x : Inport
  y : Inport  Port=2
  z : Inport  Port=3
  AddSub : xbsIndex_r3/AddSub  mode=Addition or Subtraction  precision=User Defined  arith_type="Signed  (2's comp)"  n_bits=pe_nbits  bin_pt=pe_binpt  quantization=Truncate  overflow=Wrap  latency=pipeline  explicit_period=off  period=1  en=off  dbl_ovrd=off  use_core=on  pipeline=off  use_rpm=off  gen_core=on
      settings: xl_area=[8 16 0 16 0 0 0]
  AddSub1 : xbsIndex_r3/AddSub  mode=Addition or Subtraction  precision=User Defined  arith_type="Signed  (2's comp)"  n_bits=pe_nbits  bin_pt=pe_binpt  quantization=Truncate  overflow=Wrap  latency=pipeline  explicit_period=off  period=1  en=off  dbl_ovrd=off  use_core=on  pipeline=off  use_rpm=off  gen_core=on
      settings: xl_area=[8 16 0 16 0 0 0]
  AddSub2 : xbsIndex_r3/AddSub  mode=Addition or Subtraction  precision=User Defined  arith_type="Signed  (2's comp)"  n_bits=pe_nbits  bin_pt=pe_binpt  quantization=Truncate  overflow=Wrap  latency=pipeline  explicit_period=off  period=1  en=off  dbl_ovrd=off  use_core=on  pipeline=off  use_rpm=off  gen_core=on
      settings: xl_area=[8 16 0 16 0 0 0]
  Constant : xbsIndex_r3/Constant  const=epsilon_k  arith_type="Signed  (2's comp)"  n_bits=pe_nbits  bin_pt=pe_binpt  explicit_period=off  period=1  dbl_ovrd=off
  Inverter : xbsIndex_r3/Inverter  latency=0  explicit_period=off  period=1  en=off  dbl_ovrd=off
      settings: xl_area=[1 0 0 1 0 0 0]
  Shift : xbsIndex_r3/Shift  shift_dir=Right  shift_bits=ii  precision=User Defined  arith_type="Signed  (2's comp)"  n_bits=pe_nbits  bin_pt=pe_binpt  quantization=Truncate  overflow=Wrap  latency=0  explicit_period=off  period=1  en=off  dbl_ovrd=off
      settings: xl_area=[0 0 0 0 0 0 0]
  Shift1 : xbsIndex_r3/Shift  shift_dir=Right  shift_bits=ii  precision=User Defined  arith_type="Signed  (2's comp)"  n_bits=pe_nbits  bin_pt=pe_binpt  quantization=Truncate  overflow=Wrap  latency=0  explicit_period=off  period=1  en=off  dbl_ovrd=off
      settings: xl_area=[0 0 0 0 0 0 0]
  Slice : xbsIndex_r3/Slice  mode=Upper Bit Location + Width  nbits=1  bit1=0  base1=MSB of Input  bit0=0  base0=LSB of Input  boolean_output=on  explicit_period=off  period=1  dbl_ovrd=off
  X : Outport
  Y : Outport  Port=2
  Z : Outport  Port=3
  wires:
  x/1 -> AddSub/1, Shift/1
  y/1 -> AddSub1/1, Shift1/1
  AddSub/1 -> X/1
  z/1 -> AddSub2/1, Slice/1
  AddSub1/1 -> Y/1
  AddSub2/1 -> Z/1
  Constant/1 -> AddSub2/2
  Shift/1 -> AddSub1/2
  Shift1/1 -> AddSub/2
  Slice/1 -> Inverter/1, AddSub1/3
  Inverter/1 -> AddSub2/3, AddSub/3

== system xrbsMath_r3/CORDIC SINCOS/CORDIC Fine Angle PE/CORDIC PE6 ==
  note: X = x + y if z < 0, otherwise
      |    = x - y
      | Y = y - x if z < 0, otherwise
      |    = y + x
      | Z = z + atan(1/2^i) if z < 0, otherwise
      |    = z - atan(1/2^i)
  x : Inport
  y : Inport  Port=2
  z : Inport  Port=3
  AddSub : xbsIndex_r3/AddSub  mode=Addition or Subtraction  precision=User Defined  arith_type="Signed  (2's comp)"  n_bits=pe_nbits  bin_pt=pe_binpt  quantization=Truncate  overflow=Wrap  latency=pipeline  explicit_period=off  period=1  en=off  dbl_ovrd=off  use_core=on  pipeline=off  use_rpm=off  gen_core=on
      settings: xl_area=[8 16 0 16 0 0 0]
  AddSub1 : xbsIndex_r3/AddSub  mode=Addition or Subtraction  precision=User Defined  arith_type="Signed  (2's comp)"  n_bits=pe_nbits  bin_pt=pe_binpt  quantization=Truncate  overflow=Wrap  latency=pipeline  explicit_period=off  period=1  en=off  dbl_ovrd=off  use_core=on  pipeline=off  use_rpm=off  gen_core=on
      settings: xl_area=[8 16 0 16 0 0 0]
  AddSub2 : xbsIndex_r3/AddSub  mode=Addition or Subtraction  precision=User Defined  arith_type="Signed  (2's comp)"  n_bits=pe_nbits  bin_pt=pe_binpt  quantization=Truncate  overflow=Wrap  latency=pipeline  explicit_period=off  period=1  en=off  dbl_ovrd=off  use_core=on  pipeline=off  use_rpm=off  gen_core=on
      settings: xl_area=[8 16 0 16 0 0 0]
  Constant : xbsIndex_r3/Constant  const=epsilon_k  arith_type="Signed  (2's comp)"  n_bits=pe_nbits  bin_pt=pe_binpt  explicit_period=off  period=1  dbl_ovrd=off
  Inverter : xbsIndex_r3/Inverter  latency=0  explicit_period=off  period=1  en=off  dbl_ovrd=off
      settings: xl_area=[1 0 0 1 0 0 0]
  Shift : xbsIndex_r3/Shift  shift_dir=Right  shift_bits=ii  precision=User Defined  arith_type="Signed  (2's comp)"  n_bits=pe_nbits  bin_pt=pe_binpt  quantization=Truncate  overflow=Wrap  latency=0  explicit_period=off  period=1  en=off  dbl_ovrd=off
      settings: xl_area=[0 0 0 0 0 0 0]
  Shift1 : xbsIndex_r3/Shift  shift_dir=Right  shift_bits=ii  precision=User Defined  arith_type="Signed  (2's comp)"  n_bits=pe_nbits  bin_pt=pe_binpt  quantization=Truncate  overflow=Wrap  latency=0  explicit_period=off  period=1  en=off  dbl_ovrd=off
      settings: xl_area=[0 0 0 0 0 0 0]
  Slice : xbsIndex_r3/Slice  mode=Upper Bit Location + Width  nbits=1  bit1=0  base1=MSB of Input  bit0=0  base0=LSB of Input  boolean_output=on  explicit_period=off  period=1  dbl_ovrd=off
  X : Outport
  Y : Outport  Port=2
  Z : Outport  Port=3
  wires:
  x/1 -> AddSub/1, Shift/1
  y/1 -> AddSub1/1, Shift1/1
  AddSub/1 -> X/1
  z/1 -> AddSub2/1, Slice/1
  AddSub1/1 -> Y/1
  AddSub2/1 -> Z/1
  Constant/1 -> AddSub2/2
  Shift/1 -> AddSub1/2
  Shift1/1 -> AddSub/2
  Slice/1 -> Inverter/1, AddSub1/3
  Inverter/1 -> AddSub2/3, AddSub/3

== system xrbsMath_r3/CORDIC SINCOS/CORDIC Fine Angle PE/CORDIC PE7 ==
  note: X = x + y if z < 0, otherwise
      |    = x - y
      | Y = y - x if z < 0, otherwise
      |    = y + x
      | Z = z + atan(1/2^i) if z < 0, otherwise
      |    = z - atan(1/2^i)
  x : Inport
  y : Inport  Port=2
  z : Inport  Port=3
  AddSub : xbsIndex_r3/AddSub  mode=Addition or Subtraction  precision=User Defined  arith_type="Signed  (2's comp)"  n_bits=pe_nbits  bin_pt=pe_binpt  quantization=Truncate  overflow=Wrap  latency=pipeline  explicit_period=off  period=1  en=off  dbl_ovrd=off  use_core=on  pipeline=off  use_rpm=off  gen_core=on
      settings: xl_area=[8 16 0 16 0 0 0]
  AddSub1 : xbsIndex_r3/AddSub  mode=Addition or Subtraction  precision=User Defined  arith_type="Signed  (2's comp)"  n_bits=pe_nbits  bin_pt=pe_binpt  quantization=Truncate  overflow=Wrap  latency=pipeline  explicit_period=off  period=1  en=off  dbl_ovrd=off  use_core=on  pipeline=off  use_rpm=off  gen_core=on
      settings: xl_area=[8 16 0 16 0 0 0]
  AddSub2 : xbsIndex_r3/AddSub  mode=Addition or Subtraction  precision=User Defined  arith_type="Signed  (2's comp)"  n_bits=pe_nbits  bin_pt=pe_binpt  quantization=Truncate  overflow=Wrap  latency=pipeline  explicit_period=off  period=1  en=off  dbl_ovrd=off  use_core=on  pipeline=off  use_rpm=off  gen_core=on
      settings: xl_area=[8 16 0 16 0 0 0]
  Constant : xbsIndex_r3/Constant  const=epsilon_k  arith_type="Signed  (2's comp)"  n_bits=pe_nbits  bin_pt=pe_binpt  explicit_period=off  period=1  dbl_ovrd=off
  Inverter : xbsIndex_r3/Inverter  latency=0  explicit_period=off  period=1  en=off  dbl_ovrd=off
      settings: xl_area=[1 0 0 1 0 0 0]
  Shift : xbsIndex_r3/Shift  shift_dir=Right  shift_bits=ii  precision=User Defined  arith_type="Signed  (2's comp)"  n_bits=pe_nbits  bin_pt=pe_binpt  quantization=Truncate  overflow=Wrap  latency=0  explicit_period=off  period=1  en=off  dbl_ovrd=off
      settings: xl_area=[0 0 0 0 0 0 0]
  Shift1 : xbsIndex_r3/Shift  shift_dir=Right  shift_bits=ii  precision=User Defined  arith_type="Signed  (2's comp)"  n_bits=pe_nbits  bin_pt=pe_binpt  quantization=Truncate  overflow=Wrap  latency=0  explicit_period=off  period=1  en=off  dbl_ovrd=off
      settings: xl_area=[0 0 0 0 0 0 0]
  Slice : xbsIndex_r3/Slice  mode=Upper Bit Location + Width  nbits=1  bit1=0  base1=MSB of Input  bit0=0  base0=LSB of Input  boolean_output=on  explicit_period=off  period=1  dbl_ovrd=off
  X : Outport
  Y : Outport  Port=2
  Z : Outport  Port=3
  wires:
  x/1 -> AddSub/1, Shift/1
  y/1 -> AddSub1/1, Shift1/1
  AddSub/1 -> X/1
  z/1 -> AddSub2/1, Slice/1
  AddSub1/1 -> Y/1
  AddSub2/1 -> Z/1
  Constant/1 -> AddSub2/2
  Shift/1 -> AddSub1/2
  Shift1/1 -> AddSub/2
  Slice/1 -> Inverter/1, AddSub1/3
  Inverter/1 -> AddSub2/3, AddSub/3

== system xrbsMath_r3/CORDIC SINCOS/CORDIC Fine Angle PE/CORDIC PE8 ==
  note: X = x + y if z < 0, otherwise
      |    = x - y
      | Y = y - x if z < 0, otherwise
      |    = y + x
      | Z = z + atan(1/2^i) if z < 0, otherwise
      |    = z - atan(1/2^i)
  x : Inport
  y : Inport  Port=2
  z : Inport  Port=3
  AddSub : xbsIndex_r3/AddSub  mode=Addition or Subtraction  precision=User Defined  arith_type="Signed  (2's comp)"  n_bits=pe_nbits  bin_pt=pe_binpt  quantization=Truncate  overflow=Wrap  latency=pipeline  explicit_period=off  period=1  en=off  dbl_ovrd=off  use_core=on  pipeline=off  use_rpm=off  gen_core=on
      settings: xl_area=[8 16 0 16 0 0 0]
  AddSub1 : xbsIndex_r3/AddSub  mode=Addition or Subtraction  precision=User Defined  arith_type="Signed  (2's comp)"  n_bits=pe_nbits  bin_pt=pe_binpt  quantization=Truncate  overflow=Wrap  latency=pipeline  explicit_period=off  period=1  en=off  dbl_ovrd=off  use_core=on  pipeline=off  use_rpm=off  gen_core=on
      settings: xl_area=[8 16 0 16 0 0 0]
  AddSub2 : xbsIndex_r3/AddSub  mode=Addition or Subtraction  precision=User Defined  arith_type="Signed  (2's comp)"  n_bits=pe_nbits  bin_pt=pe_binpt  quantization=Truncate  overflow=Wrap  latency=pipeline  explicit_period=off  period=1  en=off  dbl_ovrd=off  use_core=on  pipeline=off  use_rpm=off  gen_core=on
      settings: xl_area=[8 16 0 16 0 0 0]
  Constant : xbsIndex_r3/Constant  const=epsilon_k  arith_type="Signed  (2's comp)"  n_bits=pe_nbits  bin_pt=pe_binpt  explicit_period=off  period=1  dbl_ovrd=off
  Inverter : xbsIndex_r3/Inverter  latency=0  explicit_period=off  period=1  en=off  dbl_ovrd=off
      settings: xl_area=[1 0 0 1 0 0 0]
  Shift : xbsIndex_r3/Shift  shift_dir=Right  shift_bits=ii  precision=User Defined  arith_type="Signed  (2's comp)"  n_bits=pe_nbits  bin_pt=pe_binpt  quantization=Truncate  overflow=Wrap  latency=0  explicit_period=off  period=1  en=off  dbl_ovrd=off
      settings: xl_area=[0 0 0 0 0 0 0]
  Shift1 : xbsIndex_r3/Shift  shift_dir=Right  shift_bits=ii  precision=User Defined  arith_type="Signed  (2's comp)"  n_bits=pe_nbits  bin_pt=pe_binpt  quantization=Truncate  overflow=Wrap  latency=0  explicit_period=off  period=1  en=off  dbl_ovrd=off
      settings: xl_area=[0 0 0 0 0 0 0]
  Slice : xbsIndex_r3/Slice  mode=Upper Bit Location + Width  nbits=1  bit1=0  base1=MSB of Input  bit0=0  base0=LSB of Input  boolean_output=on  explicit_period=off  period=1  dbl_ovrd=off
  X : Outport
  Y : Outport  Port=2
  Z : Outport  Port=3
  wires:
  x/1 -> AddSub/1, Shift/1
  y/1 -> AddSub1/1, Shift1/1
  AddSub/1 -> X/1
  z/1 -> AddSub2/1, Slice/1
  AddSub1/1 -> Y/1
  AddSub2/1 -> Z/1
  Constant/1 -> AddSub2/2
  Shift/1 -> AddSub1/2
  Shift1/1 -> AddSub/2
  Slice/1 -> Inverter/1, AddSub1/3
  Inverter/1 -> AddSub2/3, AddSub/3

== system xrbsMath_r3/CORDIC SQRT/CORDIC Fine Angle PE/CORDIC PE1 ==
  note: X = x + y if y < 0, otherwise
      |    = x - y
      | Y = y + x if y < 0, otherwise
      |    = y - x
  x : Inport
  y : Inport  Port=2
  AddSub : xbsIndex_r3/AddSub  mode=Addition or Subtraction  precision=User Defined  arith_type="Signed  (2's comp)"  n_bits=pe_nbits  bin_pt=pe_binpt  quantization=Truncate  overflow=Wrap  latency=pipeline  explicit_period=off  period=1  en=off  dbl_ovrd=off  use_core=on  pipeline=off  use_rpm=off  gen_core=on
      settings: xl_area=[7 14 0 14 0 0 0]
  AddSub1 : xbsIndex_r3/AddSub  mode=Addition or Subtraction  precision=User Defined  arith_type="Signed  (2's comp)"  n_bits=pe_nbits  bin_pt=pe_binpt  quantization=Truncate  overflow=Wrap  latency=pipeline  explicit_period=off  period=1  en=off  dbl_ovrd=off  use_core=on  pipeline=off  use_rpm=off  gen_core=on
      settings: xl_area=[7 14 0 14 0 0 0]
  Inverter : xbsIndex_r3/Inverter  latency=0  explicit_period=off  period=1  en=off  dbl_ovrd=off
      settings: xl_area=[1 0 0 1 0 0 0]
  Shift : xbsIndex_r3/Shift  shift_dir=Right  shift_bits=ii  precision=User Defined  arith_type="Signed  (2's comp)"  n_bits=pe_nbits  bin_pt=pe_binpt  quantization=Truncate  overflow=Wrap  latency=0  explicit_period=off  period=1  en=off  dbl_ovrd=off
      settings: xl_area=[0 0 0 0 0 0 0]
  Shift1 : xbsIndex_r3/Shift  shift_dir=Right  shift_bits=ii  precision=User Defined  arith_type="Signed  (2's comp)"  n_bits=pe_nbits  bin_pt=pe_binpt  quantization=Truncate  overflow=Wrap  latency=0  explicit_period=off  period=1  en=off  dbl_ovrd=off
      settings: xl_area=[0 0 0 0 0 0 0]
  Slice : xbsIndex_r3/Slice  mode=Upper Bit Location + Width  nbits=1  bit1=0  base1=MSB of Input  bit0=0  base0=LSB of Input  boolean_output=on  explicit_period=off  period=1  dbl_ovrd=off
  X : Outport
  Y : Outport  Port=2
  wires:
  Inverter/1 -> AddSub1/3, AddSub/3
  x/1 -> AddSub/1, Shift/1
  y/1 -> AddSub1/1, Shift1/1, Slice/1
  AddSub/1 -> X/1
  AddSub1/1 -> Y/1
  Shift/1 -> AddSub1/2
  Shift1/1 -> AddSub/2
  Slice/1 -> Inverter/1

== system xrbsMath_r3/CORDIC SQRT/CORDIC Fine Angle PE/CORDIC PE10 ==
  note: X = x + y if y < 0, otherwise
      |    = x - y
      | Y = y + x if y < 0, otherwise
      |    = y - x
  x : Inport
  y : Inport  Port=2
  AddSub : xbsIndex_r3/AddSub  mode=Addition or Subtraction  precision=User Defined  arith_type="Signed  (2's comp)"  n_bits=pe_nbits  bin_pt=pe_binpt  quantization=Truncate  overflow=Wrap  latency=pipeline  explicit_period=off  period=1  en=off  dbl_ovrd=off  use_core=on  pipeline=off  use_rpm=off  gen_core=on
      settings: xl_area=[7 14 0 14 0 0 0]
  AddSub1 : xbsIndex_r3/AddSub  mode=Addition or Subtraction  precision=User Defined  arith_type="Signed  (2's comp)"  n_bits=pe_nbits  bin_pt=pe_binpt  quantization=Truncate  overflow=Wrap  latency=pipeline  explicit_period=off  period=1  en=off  dbl_ovrd=off  use_core=on  pipeline=off  use_rpm=off  gen_core=on
      settings: xl_area=[7 14 0 14 0 0 0]
  Inverter : xbsIndex_r3/Inverter  latency=0  explicit_period=off  period=1  en=off  dbl_ovrd=off
      settings: xl_area=[1 0 0 1 0 0 0]
  Shift : xbsIndex_r3/Shift  shift_dir=Right  shift_bits=ii  precision=User Defined  arith_type="Signed  (2's comp)"  n_bits=pe_nbits  bin_pt=pe_binpt  quantization=Truncate  overflow=Wrap  latency=0  explicit_period=off  period=1  en=off  dbl_ovrd=off
      settings: xl_area=[0 0 0 0 0 0 0]
  Shift1 : xbsIndex_r3/Shift  shift_dir=Right  shift_bits=ii  precision=User Defined  arith_type="Signed  (2's comp)"  n_bits=pe_nbits  bin_pt=pe_binpt  quantization=Truncate  overflow=Wrap  latency=0  explicit_period=off  period=1  en=off  dbl_ovrd=off
      settings: xl_area=[0 0 0 0 0 0 0]
  Slice : xbsIndex_r3/Slice  mode=Upper Bit Location + Width  nbits=1  bit1=0  base1=MSB of Input  bit0=0  base0=LSB of Input  boolean_output=on  explicit_period=off  period=1  dbl_ovrd=off
  X : Outport
  Y : Outport  Port=2
  wires:
  Slice/1 -> Inverter/1
  Shift1/1 -> AddSub/2
  Shift/1 -> AddSub1/2
  AddSub1/1 -> Y/1
  AddSub/1 -> X/1
  y/1 -> Slice/1, Shift1/1, AddSub1/1
  x/1 -> Shift/1, AddSub/1
  Inverter/1 -> AddSub/3, AddSub1/3

== system xrbsMath_r3/CORDIC SQRT/CORDIC Fine Angle PE/CORDIC PE11 ==
  note: X = x + y if y < 0, otherwise
      |    = x - y
      | Y = y + x if y < 0, otherwise
      |    = y - x
  x : Inport
  y : Inport  Port=2
  AddSub : xbsIndex_r3/AddSub  mode=Addition or Subtraction  precision=User Defined  arith_type="Signed  (2's comp)"  n_bits=pe_nbits  bin_pt=pe_binpt  quantization=Truncate  overflow=Wrap  latency=pipeline  explicit_period=off  period=1  en=off  dbl_ovrd=off  use_core=on  pipeline=off  use_rpm=off  gen_core=on
      settings: xl_area=[7 14 0 14 0 0 0]
  AddSub1 : xbsIndex_r3/AddSub  mode=Addition or Subtraction  precision=User Defined  arith_type="Signed  (2's comp)"  n_bits=pe_nbits  bin_pt=pe_binpt  quantization=Truncate  overflow=Wrap  latency=pipeline  explicit_period=off  period=1  en=off  dbl_ovrd=off  use_core=on  pipeline=off  use_rpm=off  gen_core=on
      settings: xl_area=[7 14 0 14 0 0 0]
  Inverter : xbsIndex_r3/Inverter  latency=0  explicit_period=off  period=1  en=off  dbl_ovrd=off
      settings: xl_area=[1 0 0 1 0 0 0]
  Shift : xbsIndex_r3/Shift  shift_dir=Right  shift_bits=ii  precision=User Defined  arith_type="Signed  (2's comp)"  n_bits=pe_nbits  bin_pt=pe_binpt  quantization=Truncate  overflow=Wrap  latency=0  explicit_period=off  period=1  en=off  dbl_ovrd=off
      settings: xl_area=[0 0 0 0 0 0 0]
  Shift1 : xbsIndex_r3/Shift  shift_dir=Right  shift_bits=ii  precision=User Defined  arith_type="Signed  (2's comp)"  n_bits=pe_nbits  bin_pt=pe_binpt  quantization=Truncate  overflow=Wrap  latency=0  explicit_period=off  period=1  en=off  dbl_ovrd=off
      settings: xl_area=[0 0 0 0 0 0 0]
  Slice : xbsIndex_r3/Slice  mode=Upper Bit Location + Width  nbits=1  bit1=0  base1=MSB of Input  bit0=0  base0=LSB of Input  boolean_output=on  explicit_period=off  period=1  dbl_ovrd=off
  X : Outport
  Y : Outport  Port=2
  wires:
  Slice/1 -> Inverter/1
  Shift1/1 -> AddSub/2
  Shift/1 -> AddSub1/2
  AddSub1/1 -> Y/1
  AddSub/1 -> X/1
  y/1 -> Slice/1, Shift1/1, AddSub1/1
  x/1 -> Shift/1, AddSub/1
  Inverter/1 -> AddSub/3, AddSub1/3

== system xrbsMath_r3/CORDIC SQRT/CORDIC Fine Angle PE/CORDIC PE12 ==
  note: X = x + y if y < 0, otherwise
      |    = x - y
      | Y = y + x if y < 0, otherwise
      |    = y - x
  x : Inport
  y : Inport  Port=2
  AddSub : xbsIndex_r3/AddSub  mode=Addition or Subtraction  precision=User Defined  arith_type="Signed  (2's comp)"  n_bits=pe_nbits  bin_pt=pe_binpt  quantization=Truncate  overflow=Wrap  latency=pipeline  explicit_period=off  period=1  en=off  dbl_ovrd=off  use_core=on  pipeline=off  use_rpm=off  gen_core=on
      settings: xl_area=[7 14 0 14 0 0 0]
  AddSub1 : xbsIndex_r3/AddSub  mode=Addition or Subtraction  precision=User Defined  arith_type="Signed  (2's comp)"  n_bits=pe_nbits  bin_pt=pe_binpt  quantization=Truncate  overflow=Wrap  latency=pipeline  explicit_period=off  period=1  en=off  dbl_ovrd=off  use_core=on  pipeline=off  use_rpm=off  gen_core=on
      settings: xl_area=[7 14 0 14 0 0 0]
  Inverter : xbsIndex_r3/Inverter  latency=0  explicit_period=off  period=1  en=off  dbl_ovrd=off
      settings: xl_area=[1 0 0 1 0 0 0]
  Shift : xbsIndex_r3/Shift  shift_dir=Right  shift_bits=ii  precision=User Defined  arith_type="Signed  (2's comp)"  n_bits=pe_nbits  bin_pt=pe_binpt  quantization=Truncate  overflow=Wrap  latency=0  explicit_period=off  period=1  en=off  dbl_ovrd=off
      settings: xl_area=[0 0 0 0 0 0 0]
  Shift1 : xbsIndex_r3/Shift  shift_dir=Right  shift_bits=ii  precision=User Defined  arith_type="Signed  (2's comp)"  n_bits=pe_nbits  bin_pt=pe_binpt  quantization=Truncate  overflow=Wrap  latency=0  explicit_period=off  period=1  en=off  dbl_ovrd=off
      settings: xl_area=[0 0 0 0 0 0 0]
  Slice : xbsIndex_r3/Slice  mode=Upper Bit Location + Width  nbits=1  bit1=0  base1=MSB of Input  bit0=0  base0=LSB of Input  boolean_output=on  explicit_period=off  period=1  dbl_ovrd=off
  X : Outport
  Y : Outport  Port=2
  wires:
  Slice/1 -> Inverter/1
  Shift1/1 -> AddSub/2
  Shift/1 -> AddSub1/2
  AddSub1/1 -> Y/1
  AddSub/1 -> X/1
  y/1 -> Slice/1, Shift1/1, AddSub1/1
  x/1 -> Shift/1, AddSub/1
  Inverter/1 -> AddSub/3, AddSub1/3
